simulink model "controlmodel"  (R2016a)
settings: Solver=ode45  StartTime=0.0  StopTime=12.0  RelTol=1e-3
values from neighbouring files (symbols this model uses):
  gainBFL = 1    [LoadModel_dampedTM.m]
  gainBFP = 1    [LoadModel_dampedTM.m]
  gainBFR = 1    [LoadModel_dampedTM.m]
  gainBFT = 1    [LoadModel_dampedTM.m]
  gainBFV = 1    [LoadModel_dampedTM.m]
  gainBFY = 1    [LoadModel_dampedTM.m]
  gainGASBF = 1    [LoadModel_dampedTM.m]
  gainGASF0 = 1    [LoadModel_dampedTM.m]
  gainGASF1 = 1    [LoadModel_dampedTM.m]
  gainGASF2 = 1    [LoadModel_dampedTM.m]
  gainGASF3 = 1    [LoadModel_dampedTM.m]
  gainIML = 1    [LoadModel_dampedTM.m]
  gainIMP = 1    [LoadModel_dampedTM.m]
  gainIMR = 1    [LoadModel_dampedTM.m]
  gainIMT = 1    [LoadModel_dampedTM.m]
  gainIMV = 1    [LoadModel_dampedTM.m]
  gainIMY = 1    [LoadModel_dampedTM.m]
  gainIPL = 1    [LoadModel_dampedTM.m]
  gainIPT = 1    [LoadModel_dampedTM.m]
  gainIPY = 1    [LoadModel_dampedTM.m]
  gainLOCK_IML = 1    [LoadModel_dampedTM.m]
  gainLOCK_IMP = 1    [LoadModel_dampedTM.m]
  gainLOCK_IMY = 1    [LoadModel_dampedTM.m]
  gainMNL = 1    [LoadModel_dampedTM.m]
  gainMNLOCK_L = 1    [LoadModel_dampedTM.m]
  gainMNLOCK_P = 1    [LoadModel_dampedTM.m]
  gainMNLOCK_Y = 1    [LoadModel_dampedTM.m]
  gainMNP = 1    [LoadModel_dampedTM.m]
  gainMNR = 1    [LoadModel_dampedTM.m]
  gainMNT = 1    [LoadModel_dampedTM.m]
  gainMNV = 1    [LoadModel_dampedTM.m]
  gainMNY = 1    [LoadModel_dampedTM.m]
  gainOL_MNP = 1    [LoadModel_dampedTM.m]
  gainOL_MNY = 1    [LoadModel_dampedTM.m]
  gainTML = 1    [LoadModel_dampedTM.m]
  gainTML_LOCK = 0    [LoadModel_dampedTM.m]
  gainTMOL_IML = 1    [LoadModel_dampedTM.m]
  gainTMOL_IMP = 1    [LoadModel_dampedTM.m]
  gainTMOL_IMY = 1    [LoadModel_dampedTM.m]
  gainTMOL_MNL = 1    [LoadModel_dampedTM.m]
  gainTMOL_MNP = 1    [LoadModel_dampedTM.m]
  gainTMOL_MNY = 1    [LoadModel_dampedTM.m]
  gainTMP = 1    [LoadModel_dampedTM.m]
  gainTMY = 1    [LoadModel_dampedTM.m]
  Kopt_angle = 0.1    [LoadModel_dampedTM.m]
  Kopt_len = 0.1    [LoadModel_dampedTM.m]
  optic = 'ETMX'    [LoadModel_dampedTM.m]
undefined symbols (not defined in the file or in its folder): cMat_BF, cMat_IM, cMat_MN, cMat_TM, Filt, gain_actBFGAS, gain_actBFL, gain_actBFP, gain_actBFR, gain_actBFT, gain_actBFV, gain_actBFY, gain_actF0GAS, gain_actF1GAS, gain_actF2GAS, gain_actF3GAS, gain_actIML, gain_actIMP, gain_actIMR, gain_actIMT, gain_actIMV, gain_actIMY, gain_actIPL, gain_actIPT, gain_actIPY, gain_actMNL, gain_actMNP, gain_actMNR, gain_actMNT, gain_actMNV, gain_actMNY, gain_actTML, gain_actTMP, gain_actTMY, SW, sys1
libraries: cstblocks x49, LiveParts x49
(part 2 of 3)

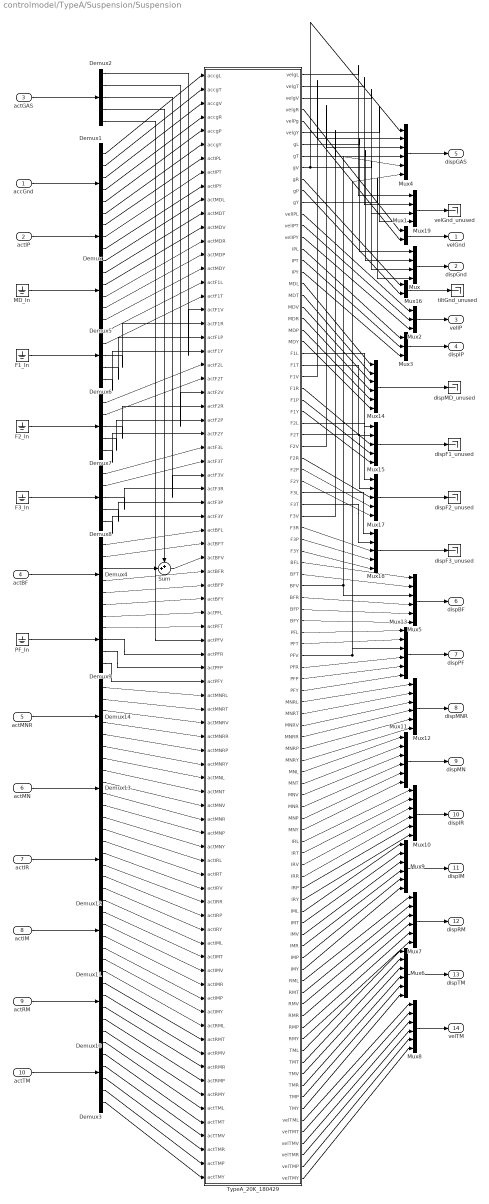
== system controlmodel/TypeA/Suspension/Suspension ==
  accGnd : Inport
  actIP : Inport  Port=2
  actGAS : Inport  Port=3
  actBF : Inport  Port=4
  actMNR : Inport  Port=5
  actMN : Inport  Port=6
  actIR : Inport  Port=7
  actIM : Inport  Port=8
  actRM : Inport  Port=9
  actTM : Inport  Port=10
  Demux : Demux  Outputs=3
  Demux{1,3..5,10..14} (9 alike) : Demux  Outputs=6
  Demux{2,6..9} (5 alike) : Demux  Outputs=5
  F1_In : Ground
  F2_In : Ground
  F3_In : Ground
  MD_In : Ground
  Mux : Mux
  Mux1 : Mux  Inputs=2
  Mux{4..14} (11 alike) : Mux  Inputs=6
  Mux15 : Mux  Inputs=5
  Mux16 : Mux  Inputs=2
  Mux17 : Mux  Inputs=5
  Mux18 : Mux  Inputs=5
  Mux19 : Mux
  Mux2 : Mux  Inputs=3
  Mux3 : Mux  Inputs=3
  PF_In : Ground
  Sum : Sum  Inputs=++|
  TypeA_20K_180429 : Subsystem
  dispF1_unused : Terminator
  dispF2_unused : Terminator
  dispF3_unused : Terminator
  dispMD_unused : Terminator
  tiltGnd_unused : Terminator
  velGnd_unused : Terminator
  velGnd : Outport
  dispGnd : Outport  Port=2
  velIP : Outport  Port=3
  dispIP : Outport  Port=4
  dispGAS : Outport  Port=5
  dispBF : Outport  Port=6
  dispPF : Outport  Port=7
  dispMNR : Outport  Port=8
  dispMN : Outport  Port=9
  dispIR : Outport  Port=10
  dispIM : Outport  Port=11
  dispRM : Outport  Port=12
  dispTM : Outport  Port=13
  velTM : Outport  Port=14
  wires:
  Mux/1 -> dispGnd/1
  Mux1/1 -> velGnd/1
  Mux2/1 -> velIP/1
  Mux3/1 -> dispIP/1
  Mux4/1 -> dispGAS/1
  Mux5/1 -> dispBF/1
  Mux6/1 -> dispTM/1
  actIP/1 -> Demux/1
  accGnd/1 -> Demux1/1
  actTM/1 -> Demux3/1
  Demux4/3 -> Sum/2
  Demux2/4 -> Sum/1
  Demux2/5 -> TypeA_20K_180429/42(actPFV)
  actBF/1 -> Demux4/1
  actGAS/1 -> Demux2/1
  Demux1/3 -> TypeA_20K_180429/3(accgV)
  Demux1/1 -> TypeA_20K_180429/1(accgL)
  Demux1/2 -> TypeA_20K_180429/2(accgT)
  Demux1/4 -> TypeA_20K_180429/4(accgR)
  Demux1/5 -> TypeA_20K_180429/5(accgP)
  Demux1/6 -> TypeA_20K_180429/6(accgY)
  Demux/1 -> TypeA_20K_180429/7(actIPL)
  Demux/2 -> TypeA_20K_180429/8(actIPT)
  Demux/3 -> TypeA_20K_180429/9(actIPY)
  MD_In/1 -> Demux5/1
  Demux5/1 -> TypeA_20K_180429/10(actMDL)
  Demux5/2 -> TypeA_20K_180429/11(actMDT)
  Demux5/3 -> TypeA_20K_180429/12(actMDV)
  Demux5/4 -> TypeA_20K_180429/13(actMDR)
  Demux5/5 -> TypeA_20K_180429/14(actMDP)
  Demux5/6 -> TypeA_20K_180429/15(actMDY)
  Demux2/1 -> TypeA_20K_180429/18(actF1V)
  Demux2/2 -> TypeA_20K_180429/24(actF2V)
  Demux2/3 -> TypeA_20K_180429/30(actF3V)
  Sum/1 -> TypeA_20K_180429/36(actBFV)
  F1_In/1 -> Demux6/1
  Demux6/2 -> TypeA_20K_180429/17(actF1T)
  Demux6/1 -> TypeA_20K_180429/16(actF1L)
  Demux6/5 -> TypeA_20K_180429/21(actF1Y)
  Demux6/3 -> TypeA_20K_180429/19(actF1R)
  Demux6/4 -> TypeA_20K_180429/20(actF1P)
  F2_In/1 -> Demux7/1
  Demux7/1 -> TypeA_20K_180429/22(actF2L)
  Demux7/2 -> TypeA_20K_180429/23(actF2T)
  Demux7/3 -> TypeA_20K_180429/25(actF2R)
  Demux7/4 -> TypeA_20K_180429/26(actF2P)
  Demux7/5 -> TypeA_20K_180429/27(actF2Y)
  F3_In/1 -> Demux8/1
  Demux8/2 -> TypeA_20K_180429/29(actF3T)
  Demux8/1 -> TypeA_20K_180429/28(actF3L)
  Demux8/5 -> TypeA_20K_180429/33(actF3Y)
  Demux8/4 -> TypeA_20K_180429/32(actF3P)
  Demux8/3 -> TypeA_20K_180429/31(actF3R)
  Demux4/1 -> TypeA_20K_180429/34(actBFL)
  Demux4/2 -> TypeA_20K_180429/35(actBFT)
  Demux4/4 -> TypeA_20K_180429/37(actBFR)
  Demux4/5 -> TypeA_20K_180429/38(actBFP)
  Demux4/6 -> TypeA_20K_180429/39(actBFY)
  PF_In/1 -> Demux9/1
  Demux9/1 -> TypeA_20K_180429/40(actPFL)
  Demux9/2 -> TypeA_20K_180429/41(actPFT)
  Demux9/4 -> TypeA_20K_180429/44(actPFP)
  Demux9/3 -> TypeA_20K_180429/43(actPFR)
  Demux9/5 -> TypeA_20K_180429/45(actPFY)
  actRM/1 -> Demux10/1
  actIM/1 -> Demux11/1
  actIR/1 -> Demux12/1
  actMN/1 -> Demux13/1
  actMNR/1 -> Demux14/1
  Demux14/4 -> TypeA_20K_180429/49(actMNRR)
  Demux14/5 -> TypeA_20K_180429/50(actMNRP)
  Demux14/6 -> TypeA_20K_180429/51(actMNRY)
  Demux14/1 -> TypeA_20K_180429/46(actMNRL)
  Demux14/2 -> TypeA_20K_180429/47(actMNRT)
  Demux14/3 -> TypeA_20K_180429/48(actMNRV)
  Demux13/2 -> TypeA_20K_180429/53(actMNT)
  Demux13/1 -> TypeA_20K_180429/52(actMNL)
  Demux13/3 -> TypeA_20K_180429/54(actMNV)
  Demux13/5 -> TypeA_20K_180429/56(actMNP)
  Demux13/4 -> TypeA_20K_180429/55(actMNR)
  Demux13/6 -> TypeA_20K_180429/57(actMNY)
  Demux12/6 -> TypeA_20K_180429/63(actIRY)
  Demux12/2 -> TypeA_20K_180429/59(actIRT)
  Demux12/5 -> TypeA_20K_180429/62(actIRP)
  Demux12/3 -> TypeA_20K_180429/60(actIRV)
  Demux12/4 -> TypeA_20K_180429/61(actIRR)
  Demux12/1 -> TypeA_20K_180429/58(actIRL)
  Demux11/2 -> TypeA_20K_180429/65(actIMT)
  Demux11/3 -> TypeA_20K_180429/66(actIMV)
  Demux11/5 -> TypeA_20K_180429/68(actIMP)
  Demux11/4 -> TypeA_20K_180429/67(actIMR)
  Demux11/1 -> TypeA_20K_180429/64(actIML)
  Demux11/6 -> TypeA_20K_180429/69(actIMY)
  Demux10/5 -> TypeA_20K_180429/74(actRMP)
  Demux10/6 -> TypeA_20K_180429/75(actRMY)
  Demux10/4 -> TypeA_20K_180429/73(actRMR)
  Demux10/3 -> TypeA_20K_180429/72(actRMV)
  Demux10/1 -> TypeA_20K_180429/70(actRML)
  Demux10/2 -> TypeA_20K_180429/71(actRMT)
  Demux3/3 -> TypeA_20K_180429/78(actTMV)
  Demux3/1 -> TypeA_20K_180429/76(actTML)
  Demux3/2 -> TypeA_20K_180429/77(actTMT)
  Demux3/4 -> TypeA_20K_180429/79(actTMR)
  Demux3/5 -> TypeA_20K_180429/80(actTMP)
  Demux3/6 -> TypeA_20K_180429/81(actTMY)
  Mux7/1 -> dispRM/1
  Mux8/1 -> velTM/1
  Mux9/1 -> dispIM/1
  Mux10/1 -> dispIR/1
  Mux11/1 -> dispMN/1
  Mux12/1 -> dispMNR/1
  Mux13/1 -> dispPF/1
  Mux14/1 -> dispMD_unused/1
  Mux15/1 -> dispF1_unused/1
  Mux16/1 -> tiltGnd_unused/1
  Mux17/1 -> dispF2_unused/1
  Mux18/1 -> dispF3_unused/1
  TypeA_20K_180429/4(velgR) -> Mux1/1
  TypeA_20K_180429/5(velPg) -> Mux1/2
  TypeA_20K_180429/8(gT) -> Mux/2
  TypeA_20K_180429/7(gL) -> Mux/1
  TypeA_20K_180429/9(gV) -> Mux/3, Mux4/1
  TypeA_20K_180429/11(gP) -> Mux16/2
  TypeA_20K_180429/10(gR) -> Mux16/1
  TypeA_20K_180429/12(gY) -> Mux/4
  TypeA_20K_180429/14(velIPT) -> Mux2/2
  TypeA_20K_180429/15(velIPY) -> Mux2/3
  TypeA_20K_180429/13(velIPL) -> Mux2/1
  TypeA_20K_180429/17(IPT) -> Mux3/2
  TypeA_20K_180429/16(IPL) -> Mux3/1
  TypeA_20K_180429/18(IPY) -> Mux3/3
  TypeA_20K_180429/19(MDL) -> Mux14/1
  TypeA_20K_180429/21(MDV) -> Mux14/3
  TypeA_20K_180429/20(MDT) -> Mux14/2
  TypeA_20K_180429/22(MDR) -> Mux14/4
  TypeA_20K_180429/23(MDP) -> Mux14/5
  TypeA_20K_180429/24(MDY) -> Mux14/6
  TypeA_20K_180429/27(F1V) -> Mux4/2
  TypeA_20K_180429/33(F2V) -> Mux4/3
  TypeA_20K_180429/39(F3V) -> Mux4/4
  TypeA_20K_180429/45(BFV) -> Mux4/5, Mux5/3
  TypeA_20K_180429/51(PFV) -> Mux4/6, Mux13/3
  TypeA_20K_180429/25(F1L) -> Mux15/1
  TypeA_20K_180429/26(F1T) -> Mux15/2
  TypeA_20K_180429/30(F1Y) -> Mux15/5
  TypeA_20K_180429/28(F1R) -> Mux15/3
  TypeA_20K_180429/29(F1P) -> Mux15/4
  TypeA_20K_180429/31(F2L) -> Mux17/1
  TypeA_20K_180429/32(F2T) -> Mux17/2
  TypeA_20K_180429/34(F2R) -> Mux17/3
  TypeA_20K_180429/36(F2Y) -> Mux17/5
  TypeA_20K_180429/35(F2P) -> Mux17/4
  TypeA_20K_180429/37(F3L) -> Mux18/1
  TypeA_20K_180429/38(F3T) -> Mux18/2
  TypeA_20K_180429/42(F3Y) -> Mux18/5
  TypeA_20K_180429/41(F3P) -> Mux18/4
  TypeA_20K_180429/40(F3R) -> Mux18/3
  TypeA_20K_180429/47(BFP) -> Mux5/5
  TypeA_20K_180429/48(BFY) -> Mux5/6
  TypeA_20K_180429/46(BFR) -> Mux5/4
  TypeA_20K_180429/44(BFT) -> Mux5/2
  TypeA_20K_180429/43(BFL) -> Mux5/1
  TypeA_20K_180429/54(PFY) -> Mux13/6
  TypeA_20K_180429/49(PFL) -> Mux13/1
  TypeA_20K_180429/50(PFT) -> Mux13/2
  TypeA_20K_180429/52(PFR) -> Mux13/4
  TypeA_20K_180429/53(PFP) -> Mux13/5
  TypeA_20K_180429/56(MNRT) -> Mux12/2
  TypeA_20K_180429/60(MNRY) -> Mux12/6
  TypeA_20K_180429/57(MNRV) -> Mux12/3
  TypeA_20K_180429/58(MNRR) -> Mux12/4
  TypeA_20K_180429/55(MNRL) -> Mux12/1
  TypeA_20K_180429/59(MNRP) -> Mux12/5
  TypeA_20K_180429/64(MNR) -> Mux11/4
  TypeA_20K_180429/61(MNL) -> Mux11/1
  TypeA_20K_180429/63(MNV) -> Mux11/3
  TypeA_20K_180429/62(MNT) -> Mux11/2
  TypeA_20K_180429/66(MNY) -> Mux11/6
  TypeA_20K_180429/65(MNP) -> Mux11/5
  TypeA_20K_180429/71(IRP) -> Mux10/5
  TypeA_20K_180429/69(IRV) -> Mux10/3
  TypeA_20K_180429/72(IRY) -> Mux10/6
  TypeA_20K_180429/70(IRR) -> Mux10/4
  TypeA_20K_180429/68(IRT) -> Mux10/2
  TypeA_20K_180429/67(IRL) -> Mux10/1
  TypeA_20K_180429/73(IML) -> Mux9/1
  TypeA_20K_180429/75(IMV) -> Mux9/3
  TypeA_20K_180429/74(IMT) -> Mux9/2
  TypeA_20K_180429/76(IMR) -> Mux9/4
  TypeA_20K_180429/77(IMP) -> Mux9/5
  TypeA_20K_180429/78(IMY) -> Mux9/6
  TypeA_20K_180429/83(RMP) -> Mux7/5
  TypeA_20K_180429/84(RMY) -> Mux7/6
  TypeA_20K_180429/79(RML) -> Mux7/1
  TypeA_20K_180429/81(RMV) -> Mux7/3
  TypeA_20K_180429/80(RMT) -> Mux7/2
  TypeA_20K_180429/82(RMR) -> Mux7/4
  TypeA_20K_180429/85(TML) -> Mux6/1
  TypeA_20K_180429/86(TMT) -> Mux6/2
  TypeA_20K_180429/88(TMR) -> Mux6/4
  TypeA_20K_180429/87(TMV) -> Mux6/3
  TypeA_20K_180429/89(TMP) -> Mux6/5
  TypeA_20K_180429/90(TMY) -> Mux6/6
  TypeA_20K_180429/93(velTMV) -> Mux8/3
  TypeA_20K_180429/94(velTMR) -> Mux8/4
  TypeA_20K_180429/96(velTMY) -> Mux8/6
  TypeA_20K_180429/91(velTML) -> Mux8/1
  TypeA_20K_180429/95(velTMP) -> Mux8/5
  TypeA_20K_180429/92(velTMT) -> Mux8/2
  Mux19/1 -> velGnd_unused/1
  TypeA_20K_180429/1(velgL) -> Mux19/1
  TypeA_20K_180429/2(velgT) -> Mux19/2
  TypeA_20K_180429/3(velgV) -> Mux19/3
  TypeA_20K_180429/6(velgY) -> Mux19/4

== system controlmodel/TypeA/Suspension/aMatrix_BF ==
  aMat_in : Inport
  cMat_BF : Constant  Value=cMat_BF  VectorParams1D=off
  coupling_BF : Product  Multiplication=Matrix(*)
  actBF : Outport
  wires:
  coupling_BF/1 -> actBF/1
  aMat_in/1 -> coupling_BF/2
  cMat_BF/1 -> coupling_BF/1

== system controlmodel/TypeA/Suspension/aMatrix_GAS ==
  aMat_in : Inport
  Add{1..4} (4 alike) : Sum  Inputs=+-
  Demux4 : Demux  Outputs=5
  Mux3 : Mux  Inputs=5
  actGAS : Outport
  wires:
  aMat_in/1 -> Demux4/1
  Mux3/1 -> actGAS/1
  Add1/1 -> Mux3/1
  Add2/1 -> Mux3/2
  Demux4/3 -> Add3/1, Add2/2
  Demux4/2 -> Add1/2, Add2/1
  Demux4/1 -> Add1/1
  Demux4/5 -> Mux3/5, Add4/2
  Add4/1 -> Mux3/4
  Add3/1 -> Mux3/3
  Demux4/4 -> Add3/2, Add4/1

== system controlmodel/TypeA/Suspension/aMatrix_IM ==
  aMat_in : Inport
  Gain : Gain  Gain=-1
  cMat_IM : Constant  Value=cMat_IM  VectorParams1D=off
  coupling_IM : Product  Multiplication=Matrix(*)
  actIR : Outport
  actIM : Outport  Port=2
  wires:
  coupling_IM/1 -> actIM/1, Gain/1
  aMat_in/1 -> coupling_IM/2
  cMat_IM/1 -> coupling_IM/1
  Gain/1 -> actIR/1

== system controlmodel/TypeA/Suspension/aMatrix_MN ==
  aMat_in : Inport
  Gain : Gain  Gain=-1
  cMat_MN : Constant  Value=cMat_MN  VectorParams1D=off
  coupling_MN : Product  Multiplication=Matrix(*)
  actMNR : Outport
  actMN : Outport  Port=2
  wires:
  coupling_MN/1 -> actMN/1, Gain/1
  aMat_in/1 -> coupling_MN/2
  cMat_MN/1 -> coupling_MN/1
  Gain/1 -> actMNR/1

== system controlmodel/TypeA/Suspension/aMatrix_TM ==
  aMat_in : Inport
  Demux : Demux  Outputs=3
  Demux1 : Demux  Outputs=3
  Gain : Gain  Gain=-1
  Ground{,1..5} (6 alike) : Ground
  Mux : Mux  Inputs=6
  Mux1 : Mux  Inputs=6
  cMat_TM : Constant  Value=cMat_TM  VectorParams1D=off
  coupling_TM : Product  Multiplication=Matrix(*)
  actRM : Outport
  actTM : Outport  Port=2
  wires:
  coupling_TM/1 -> Demux1/1, Gain/1
  aMat_in/1 -> coupling_TM/2  "3DoF"
  cMat_TM/1 -> coupling_TM/1
  Gain/1 -> Demux/1
  Demux/1 -> Mux/1
  Demux/2 -> Mux/5
  Demux/3 -> Mux/6
  Demux1/1 -> Mux1/1
  Demux1/3 -> Mux1/6
  Demux1/2 -> Mux1/5
  Ground/1 -> Mux/2
  Ground1/1 -> Mux/3
  Ground2/1 -> Mux/4
  Ground4/1 -> Mux1/3
  Ground3/1 -> Mux1/2
  Ground5/1 -> Mux1/4
  Mux/1 -> actRM/1  "6DoF"
  Mux1/1 -> actTM/1  "6DoF"

== system controlmodel/TypeA/Suspension/sMatrix_BF_LVDT ==
  dispGnd : Inport
  dispBF : Inport  Port=2
  Add2 : Sum  Inputs=-+
  Demux : Demux
  Ground : Ground
  Ground1 : Ground
  Mux : Mux  Inputs=6
  BF_LVDT : Outport
  wires:
  Add2/1 -> BF_LVDT/1  "6DoF"
  dispBF/1 -> Add2/2  "6DoF"
  dispGnd/1 -> Demux/1  "4DoF"
  Demux/1 -> Mux/1  "L"
  Demux/2 -> Mux/2  "T"
  Demux/3 -> Mux/3  "V"
  Demux/4 -> Mux/6  "Y"
  Ground/1 -> Mux/4  "R"
  Ground1/1 -> Mux/5  "P"
  Mux/1 -> Add2/1

== system controlmodel/TypeA/Suspension/sMatrix_GAS_LVDT ==
  dispGAS : Inport
  Add{1..5} (5 alike) : Sum  Inputs=-+
  Demux4 : Demux  Outputs=6
  Mux3 : Mux  Inputs=5
  GAS_LVDT : Outport
  wires:
  dispGAS/1 -> Demux4/1
  Demux4/1 -> Add2/1  "VGnd = IPV"
  Demux4/2 -> Add1/1, Add2/2  "VF1"
  Demux4/3 -> Add1/2, Add3/1  "VF2"
  Demux4/4 -> Add4/1, Add3/2  "VF3"
  Add2/1 -> Mux3/1  "GASF0"
  Add1/1 -> Mux3/2  "GASF1"
  Add3/1 -> Mux3/3  "GASF2"
  Mux3/1 -> GAS_LVDT/1
  Demux4/5 -> Add5/1, Add4/2  "VBF"
  Demux4/6 -> Add5/2  "VPF"
  Add4/1 -> Mux3/4  "GASF3"
  Add5/1 -> Mux3/5  "GASBF"

== system controlmodel/TypeA/Suspension/sMatrix_IM_PS ==
  dispIR : Inport
  dispIM : Inport  Port=2
  Add2 : Sum  Inputs=-+
  IM_PS : Outport
  wires:
  Add2/1 -> IM_PS/1
  dispIM/1 -> Add2/2
  dispIR/1 -> Add2/1

== system controlmodel/TypeA/Suspension/sMatrix_IP_LVDT ==
  dispGnd : Inport
  dispIP : Inport  Port=2
  Add2 : Sum  Inputs=-+
  Demux : Demux
  Mux : Mux  Inputs=3
  Terminator : Terminator
  IP_LVDT : Outport
  wires:
  Add2/1 -> IP_LVDT/1
  dispIP/1 -> Add2/2
  dispGnd/1 -> Demux/1
  Demux/1 -> Mux/1  "L"
  Demux/2 -> Mux/2  "T"
  Demux/4 -> Mux/3  "Y"
  Demux/3 -> Terminator/1  "V"
  Mux/1 -> Add2/1

== system controlmodel/TypeA/Suspension/sMatrix_MN_OpLev ==
  dispMN : Inport
  Demux4 : Demux  Outputs=6
  Mux3 : Mux  Inputs=3
  dispMNL : Terminator
  dispMNT : Terminator
  dispMNV : Terminator
  MN_OpLev : Outport
  wires:
  dispMN/1 -> Demux4/1
  Mux3/1 -> MN_OpLev/1
  Demux4/1 -> dispMNL/1
  Demux4/2 -> dispMNT/1
  Demux4/3 -> dispMNV/1
  Demux4/4 -> Mux3/1
  Demux4/5 -> Mux3/2
  Demux4/6 -> Mux3/3

== system controlmodel/TypeA/Suspension/sMatrix_MN_PS ==
  dispMNR : Inport
  dispMN : Inport  Port=2
  Add2 : Sum  Inputs=-+
  MN_PS : Outport
  wires:
  Add2/1 -> MN_PS/1
  dispMN/1 -> Add2/2
  dispMNR/1 -> Add2/1

== system controlmodel/TypeA/Suspension/sMatrix_PF_OpLev ==
  dispPF : Inport
  Demux4 : Demux  Outputs=6
  Mux3 : Mux  Inputs=3
  dispLPF : Terminator
  dispTPF : Terminator
  dispVPF : Terminator
  OpLev_PF : Outport
  wires:
  dispPF/1 -> Demux4/1
  Mux3/1 -> OpLev_PF/1
  Demux4/1 -> dispLPF/1
  Demux4/2 -> dispTPF/1
  Demux4/3 -> dispVPF/1
  Demux4/4 -> Mux3/1
  Demux4/5 -> Mux3/2
  Demux4/6 -> Mux3/3

== system controlmodel/TypeA/Suspension/sMatrix_TM_OpLev ==
  dispTM : Inport
  dispGND : Inport  Port=2
  Add : Sum  Inputs=-+
  Demux : Demux
  Demux4 : Demux  Outputs=6
  Mux3 : Mux  Inputs=3
  dispTMR : Terminator
  dispTMT{,1..3} (4 alike) : Terminator
  dispTMV : Terminator
  TM_OpLev : Outport
  wires:
  dispTM/1 -> Demux4/1
  Mux3/1 -> TM_OpLev/1
  Demux4/2 -> dispTMT/1
  Demux4/3 -> dispTMV/1
  Demux4/4 -> dispTMR/1
  Demux4/5 -> Mux3/2
  Demux4/6 -> Mux3/3
  Demux/1 -> Add/1
  dispGND/1 -> Demux/1
  Demux/2 -> dispTMT1/1
  Demux/3 -> dispTMT2/1
  Demux/4 -> dispTMT3/1
  Demux4/1 -> Add/2
  Add/1 -> Mux3/1

== system controlmodel/TypeA/Suspension/sMatrix_TM_PS ==
  dispRM : Inport
  dispTM : Inport  Port=2
  Add2 : Sum  Inputs=-+
  Demux : Demux  Outputs=6
  Demux1 : Demux  Outputs=6
  Mux : Mux  Inputs=3
  Mux1 : Mux  Inputs=3
  Terminator{,1..5} (6 alike) : Terminator
  TM_PS : Outport
  wires:
  Add2/1 -> TM_PS/1  "(L, P, Y)"
  dispRM/1 -> Demux/1
  dispTM/1 -> Demux1/1
  Demux/1 -> Mux/1  "L"
  Demux/5 -> Mux/2  "P"
  Demux/6 -> Mux/3  "Y"
  Demux1/1 -> Mux1/1  "L"
  Demux1/5 -> Mux1/2  "P"
  Demux1/6 -> Mux1/3  "Y"
  Mux/1 -> Add2/1
  Mux1/1 -> Add2/2
  Demux/2 -> Terminator/1  "T"
  Demux/4 -> Terminator2/1  "R"
  Demux/3 -> Terminator1/1  "V"
  Demux1/4 -> Terminator5/1  "R"
  Demux1/2 -> Terminator3/1  "T"
  Demux1/3 -> Terminator4/1  "V"

== system controlmodel/TypeA/Controller/BFservo/Servo_LBF ==
  In : Inport
  BF_DAMP_L : cstblocks/LTI System  sys=Filt('BF_DAMP_L')  IC=[]
  K1:VIS-OPTIC_BF_DAMP_L : LiveParts/LiveFilter  Tag=LiveFilter  par=Filt_BF_DAMP_L  prefix=['K1:VIS-',optic,'_BF_DAMP_L']  site='kamioka'  feModel=['K1VIS',optic,'T']  fmName=[optic,'_BF_DAMP_L']  flexTf=on  viewGui=off
      settings: AttributesFormatString=%<Tag>
  Out : Outport
  wires:
  In/1 -> BF_DAMP_L/1
  BF_DAMP_L/1 -> Out/1

== system controlmodel/TypeA/Controller/BFservo/Servo_PBF ==
  In : Inport
  BF_DAMP_P : cstblocks/LTI System  sys=Filt('BF_DAMP_P')  IC=[]
  K1:VIS-OPTIC_BF_DAMP_P : LiveParts/LiveFilter  Tag=LiveFilter  par=Filt_BF_DAMP_P  prefix=['K1:VIS-',optic,'_BF_DAMP_P']  site='kamioka'  feModel=['K1VIS',optic,'T']  fmName=[optic,'_BF_DAMP_P']  flexTf=on  viewGui=off
      settings: AttributesFormatString=%<Tag>
  Out : Outport
  wires:
  In/1 -> BF_DAMP_P/1
  BF_DAMP_P/1 -> Out/1

== system controlmodel/TypeA/Controller/BFservo/Servo_RBF ==
  In : Inport
  BF_DAMP_R : cstblocks/LTI System  sys=Filt('BF_DAMP_R')  IC=[]
  K1:VIS-OPTIC_BF_DAMP_R : LiveParts/LiveFilter  Tag=LiveFilter  par=Filt_BF_DAMP_R  prefix=['K1:VIS-',optic,'_BF_DAMP_R']  site='kamioka'  feModel=['K1VIS',optic,'T']  fmName=[optic,'_BF_DAMP_R']  flexTf=on  viewGui=off
      settings: AttributesFormatString=%<Tag>
  Out : Outport
  wires:
  In/1 -> BF_DAMP_R/1
  BF_DAMP_R/1 -> Out/1

== system controlmodel/TypeA/Controller/BFservo/Servo_TBF ==
  In : Inport
  BF_DAMP_T : cstblocks/LTI System  sys=Filt('BF_DAMP_T')  IC=[]
  K1:VIS-OPTIC_BF_DAMP_T : LiveParts/LiveFilter  Tag=LiveFilter  par=Filt_BF_DAMP_T  prefix=['K1:VIS-',optic,'_BF_DAMP_T']  site='kamioka'  feModel=['K1VIS',optic,'T']  fmName=[optic,'_BF_DAMP_T']  flexTf=on  viewGui=off
      settings: AttributesFormatString=%<Tag>
  Out : Outport
  wires:
  In/1 -> BF_DAMP_T/1
  BF_DAMP_T/1 -> Out/1

== system controlmodel/TypeA/Controller/BFservo/Servo_VBF ==
  In : Inport
  BF_DAMP_V : cstblocks/LTI System  sys=Filt('BF_DAMP_V')  IC=[]
  K1:VIS-OPTIC_BF_DAMP_V : LiveParts/LiveFilter  Tag=LiveFilter  par=Filt_BF_DAMP_V  prefix=['K1:VIS-',optic,'_BF_DAMP_V']  site='kamioka'  feModel=['K1VIS',optic,'T']  fmName=[optic,'_BF_DAMP_V']  flexTf=on  viewGui=off
      settings: AttributesFormatString=%<Tag>
  Out : Outport
  wires:
  In/1 -> BF_DAMP_V/1
  BF_DAMP_V/1 -> Out/1

== system controlmodel/TypeA/Controller/BFservo/Servo_YBF ==
  In : Inport
  BF_DAMP_Y : cstblocks/LTI System  sys=Filt('BF_DAMP_Y')  IC=[]
  K1:VIS-OPTIC_BF_DAMP_Y : LiveParts/LiveFilter  Tag=LiveFilter  par=Filt_BF_DAMP_Y  prefix=['K1:VIS-',optic,'_BF_DAMP_Y']  site='kamioka'  feModel=['K1VIS',optic,'T']  fmName=[optic,'_BF_DAMP_Y']  flexTf=on  viewGui=off
      settings: AttributesFormatString=%<Tag>
  Out : Outport
  wires:
  In/1 -> BF_DAMP_Y/1
  BF_DAMP_Y/1 -> Out/1

== system controlmodel/TypeA/Controller/GASservo/Servo_GASBF ==
  In : Inport
  BF_DAMP_GAS : cstblocks/LTI System  sys=Filt('BF_DAMP_GAS')  IC=[]
  K1:VIS-OPTIC_BF_DAMP_GAS : LiveParts/LiveFilter  Tag=LiveFilter  par=Filt_BF_DAMP_GAS  prefix=['K1:VIS-',optic,'_BF_DAMP_GAS']  site='kamioka'  feModel=['K1VIS',optic,'T']  fmName=[optic,'_BF_DAMP_GAS']  flexTf=on  viewGui=off
      settings: AttributesFormatString=%<Tag>
  Out : Outport
  wires:
  In/1 -> BF_DAMP_GAS/1
  BF_DAMP_GAS/1 -> Out/1

== system controlmodel/TypeA/Controller/GASservo/Servo_GASF0 ==
  In : Inport
  F0_DAMP_GAS : cstblocks/LTI System  sys=Filt('F0_DAMP_GAS')  IC=[]
  K1:VIS-OPTIC_F0_DAMP_GAS : LiveParts/LiveFilter  Tag=LiveFilter  par=Filt_F0_DAMP_GAS  prefix=['K1:VIS-',optic,'_F0_DAMP_GAS']  site='kamioka'  feModel=['K1VIS',optic,'T']  fmName=[optic,'_F0_DAMP_GAS']  flexTf=on  viewGui=off
      settings: AttributesFormatString=%<Tag>
  Out : Outport
  wires:
  In/1 -> F0_DAMP_GAS/1
  F0_DAMP_GAS/1 -> Out/1

== system controlmodel/TypeA/Controller/GASservo/Servo_GASF1 ==
  In : Inport
  F1_DAMP_GAS : cstblocks/LTI System  sys=Filt('F1_DAMP_GAS')  IC=[]
  K1:VIS-OPTIC_F1_DAMP_GAS : LiveParts/LiveFilter  Tag=LiveFilter  par=Filt_F1_DAMP_GAS  prefix=['K1:VIS-',optic,'_F1_DAMP_GAS']  site='kamioka'  feModel=['K1VIS',optic,'T']  fmName=[optic,'_F1_DAMP_GAS']  flexTf=on  viewGui=off
      settings: AttributesFormatString=%<Tag>
  Out : Outport
  wires:
  In/1 -> F1_DAMP_GAS/1
  F1_DAMP_GAS/1 -> Out/1

== system controlmodel/TypeA/Controller/GASservo/Servo_GASF2 ==
  In : Inport
  F2_DAMP_GAS : cstblocks/LTI System  sys=Filt('F2_DAMP_GAS')  IC=[]
  K1:VIS-OPTIC_F2_DAMP_GAS : LiveParts/LiveFilter  Tag=LiveFilter  par=Filt_F2_DAMP_GAS  prefix=['K1:VIS-',optic,'_F2_DAMP_GAS']  site='kamioka'  feModel=['K1VIS',optic,'T']  fmName=[optic,'_F2_DAMP_GAS']  flexTf=on  viewGui=off
      settings: AttributesFormatString=%<Tag>
  Out : Outport
  wires:
  In/1 -> F2_DAMP_GAS/1
  F2_DAMP_GAS/1 -> Out/1

== system controlmodel/TypeA/Controller/GASservo/Servo_GASF3 ==
  In : Inport
  F3_DAMP_GAS : cstblocks/LTI System  sys=Filt('F3_DAMP_GAS')  IC=[]
  K1:VIS-OPTIC_F3_DAMP_GAS : LiveParts/LiveFilter  Tag=LiveFilter  par=Filt_F3_DAMP_GAS  prefix=['K1:VIS-',optic,'_F3_DAMP_GAS']  site='kamioka'  feModel=['K1VIS',optic,'T']  fmName=[optic,'_F3_DAMP_GAS']  flexTf=on  viewGui=off
      settings: AttributesFormatString=%<Tag>
  Out : Outport
  wires:
  In/1 -> F3_DAMP_GAS/1
  F3_DAMP_GAS/1 -> Out/1

== system controlmodel/TypeA/Controller/IMservo/Damp_LIM ==
  In : Inport
  IM_PSDAMP_L : cstblocks/LTI System  sys=Filt('IM_PSDAMP_L')  IC=[]
  K1:VIS-OPTIC_IM_PSDAMP_L : LiveParts/LiveFilter  Tag=LiveFilter  par=Filt_IM_PSDAMP_L  prefix=['K1:VIS-',optic,'_IM_PSDAMP_L']  site='kamioka'  feModel=['K1VIS',optic,'P']  fmName=[optic,'_IM_PSDAMP_L']  flexTf=on  viewGui=off
      settings: AttributesFormatString=%<Tag>
  Out : Outport
  wires:
  In/1 -> IM_PSDAMP_L/1
  IM_PSDAMP_L/1 -> Out/1

== system controlmodel/TypeA/Controller/IMservo/Damp_PIM ==
  In : Inport
  IM_PSDAMP_P : cstblocks/LTI System  sys=Filt('IM_PSDAMP_P')  IC=[]
  K1:VIS-OPTIC_IM_PSDAMP_P : LiveParts/LiveFilter  Tag=LiveFilter  par=Filt_IM_PSDAMP_P  prefix=['K1:VIS-',optic,'_IM_PSDAMP_P']  site='kamioka'  feModel=['K1VIS',optic,'P']  fmName=[optic,'_IM_PSDAMP_P']  flexTf=on  viewGui=off
      settings: AttributesFormatString=%<Tag>
  Out : Outport
  wires:
  In/1 -> IM_PSDAMP_P/1
  IM_PSDAMP_P/1 -> Out/1

== system controlmodel/TypeA/Controller/IMservo/Damp_RIM ==
  In : Inport
  IM_PSDAMP_R : cstblocks/LTI System  sys=Filt('IM_PSDAMP_R')  IC=[]
  K1:VIS-OPTIC_IM_PSDAMP_R : LiveParts/LiveFilter  Tag=LiveFilter  par=Filt_IM_PSDAMP_R  prefix=['K1:VIS-',optic,'_IM_PSDAMP_R']  site='kamioka'  feModel=['K1VIS',optic,'P']  fmName=[optic,'_IM_PSDAMP_R']  flexTf=on  viewGui=off
      settings: AttributesFormatString=%<Tag>
  Out : Outport
  wires:
  In/1 -> IM_PSDAMP_R/1
  IM_PSDAMP_R/1 -> Out/1

== system controlmodel/TypeA/Controller/IMservo/Damp_TIM ==
  In : Inport
  IM_PSDAMP_T : cstblocks/LTI System  sys=Filt('IM_PSDAMP_T')  IC=[]
  K1:VIS-OPTIC_IM_PSDAMP_T : LiveParts/LiveFilter  Tag=LiveFilter  par=Filt_IM_PSDAMP_T  prefix=['K1:VIS-',optic,'_IM_PSDAMP_T']  site='kamioka'  feModel=['K1VIS',optic,'P']  fmName=[optic,'_IM_PSDAMP_T']  flexTf=on  viewGui=off
      settings: AttributesFormatString=%<Tag>
  Out : Outport
  wires:
  In/1 -> IM_PSDAMP_T/1
  IM_PSDAMP_T/1 -> Out/1

== system controlmodel/TypeA/Controller/IMservo/Damp_VIM ==
  In : Inport
  IM_PSDAMP_V : cstblocks/LTI System  sys=Filt('IM_PSDAMP_V')  IC=[]
  K1:VIS-OPTIC_IM_PSDAMP_V : LiveParts/LiveFilter  Tag=LiveFilter  par=Filt_IM_PSDAMP_V  prefix=['K1:VIS-',optic,'_IM_PSDAMP_V']  site='kamioka'  feModel=['K1VIS',optic,'P']  fmName=[optic,'_IM_PSDAMP_V']  flexTf=on  viewGui=off
      settings: AttributesFormatString=%<Tag>
  Out : Outport
  wires:
  In/1 -> IM_PSDAMP_V/1
  IM_PSDAMP_V/1 -> Out/1

== system controlmodel/TypeA/Controller/IMservo/Damp_YIM ==
  In : Inport
  IM_PSDAMP_Y : cstblocks/LTI System  sys=Filt('IM_PSDAMP_Y')  IC=[]
  K1:VIS-OPTIC_IM_PSDAMP_Y : LiveParts/LiveFilter  Tag=LiveFilter  par=Filt_IM_PSDAMP_Y  prefix=['K1:VIS-',optic,'_IM_PSDAMP_Y']  site='kamioka'  feModel=['K1VIS',optic,'P']  fmName=[optic,'_IM_PSDAMP_Y']  flexTf=on  viewGui=off
      settings: AttributesFormatString=%<Tag>
  Out : Outport
  wires:
  In/1 -> IM_PSDAMP_Y/1
  IM_PSDAMP_Y/1 -> Out/1

== system controlmodel/TypeA/Controller/IMservo/IMLOCK_L ==
  In : Inport
  IM_LOCK_L : cstblocks/LTI System  sys=Filt('IM_LOCK_L')  IC=[]
  K1:VIS-OPTIC_IM_LOCK_L : LiveParts/LiveFilter  Tag=LiveFilter  par=Filt_IM_LOCK_L  prefix=['K1:VIS-',optic,'_IM_LOCK_L']  site='kamioka'  feModel=['K1VIS',optic,'P']  fmName=[optic,'_IM_LOCK_L']  flexTf=on  viewGui=off
      settings: AttributesFormatString=%<Tag>
  Out : Outport
  wires:
  In/1 -> IM_LOCK_L/1
  IM_LOCK_L/1 -> Out/1

== system controlmodel/TypeA/Controller/IMservo/IMLOCK_P ==
  In : Inport
  IM_LOCK_P : cstblocks/LTI System  sys=Filt('IM_LOCK_P')  IC=[]
  K1:VIS-OPTIC_IM_LOCK_P : LiveParts/LiveFilter  Tag=LiveFilter  par=Filt_IM_LOCK_P  prefix=['K1:VIS-',optic,'_IM_LOCK_P']  site='kamioka'  feModel=['K1VIS',optic,'P']  fmName=[optic,'_IM_LOCK_P']  flexTf=on  viewGui=off
      settings: AttributesFormatString=%<Tag>
  Out : Outport
  wires:
  In/1 -> IM_LOCK_P/1
  IM_LOCK_P/1 -> Out/1

== system controlmodel/TypeA/Controller/IMservo/IMLOCK_Y ==
  In : Inport
  IM_LOCK_Y : cstblocks/LTI System  sys=Filt('IM_LOCK_Y')  IC=[]
  K1:VIS-OPTIC_IM_LOCK_Y : LiveParts/LiveFilter  Tag=LiveFilter  par=Filt_IM_LOCK_Y  prefix=['K1:VIS-',optic,'_IM_LOCK_Y']  site='kamioka'  feModel=['K1VIS',optic,'P']  fmName=[optic,'_IM_LOCK_Y']  flexTf=on  viewGui=off
      settings: AttributesFormatString=%<Tag>
  Out : Outport
  wires:
  In/1 -> IM_LOCK_Y/1
  IM_LOCK_Y/1 -> Out/1

== system controlmodel/TypeA/Controller/IMservo/TMOLDamp_LIM ==
  In : Inport
  IM_TMOLDAMP_L : cstblocks/LTI System  sys=Filt('IM_TMOLDAMP_L')  IC=[]
  K1:VIS-OPTIC_IM_TMOLDAMP_L : LiveParts/LiveFilter  Tag=LiveFilter  par=Filt_IM_TMOLDAMP_L  prefix=['K1:VIS-',optic,'_IM_TMOLDAMP_L']  site='kamioka'  feModel=['K1VIS',optic,'P']  fmName=[optic,'_IM_TMOLDAMP_L']  flexTf=on  viewGui=off
      settings: AttributesFormatString=%<Tag>
  Out : Outport
  wires:
  In/1 -> IM_TMOLDAMP_L/1
  IM_TMOLDAMP_L/1 -> Out/1

== system controlmodel/TypeA/Controller/IMservo/TMOLDamp_PIM ==
  In : Inport
  IM_TMOLDAMP_P : cstblocks/LTI System  sys=Filt('IM_TMOLDAMP_P')  IC=[]
  K1:VIS-OPTIC_IM_TMOLDAMP_P : LiveParts/LiveFilter  Tag=LiveFilter  par=Filt_IM_TMOLDAMP_P  prefix=['K1:VIS-',optic,'_IM_TMOLDAMP_P']  site='kamioka'  feModel=['K1VIS',optic,'P']  fmName=[optic,'_IM_TMOLDAMP_P']  flexTf=on  viewGui=off
      settings: AttributesFormatString=%<Tag>
  Out : Outport
  wires:
  In/1 -> IM_TMOLDAMP_P/1
  IM_TMOLDAMP_P/1 -> Out/1

== system controlmodel/TypeA/Controller/IMservo/TMOLDamp_YIM ==
  In : Inport
  IM_TMOLDAMP_Y : cstblocks/LTI System  sys=Filt('IM_TMOLDAMP_Y')  IC=[]
  K1:VIS-OPTIC_IM_TMOLDAMP_Y : LiveParts/LiveFilter  Tag=LiveFilter  par=Filt_IM_TMOLDAMP_Y  prefix=['K1:VIS-',optic,'_IM_TMOLDAMP_Y']  site='kamioka'  feModel=['K1VIS',optic,'P']  fmName=[optic,'_IM_TMOLDAMP_Y']  flexTf=on  viewGui=off
      settings: AttributesFormatString=%<Tag>
  Out : Outport
  wires:
  In/1 -> IM_TMOLDAMP_Y/1
  IM_TMOLDAMP_Y/1 -> Out/1

== system controlmodel/TypeA/Controller/IPservo/Servo_LIP ==
  In : Inport
  IP_DAMP_L : cstblocks/LTI System  sys=Filt('IP_DAMP_L')  IC=[]
  K1:VIS-OPTIC_IP_DAMP_L : LiveParts/LiveFilter  Tag=LiveFilter  par=Filt_IP_DAMP_L  prefix=['K1:VIS-',optic,'_IP_DAMP_L']  site='kamioka'  feModel=['K1VIS',optic,'T']  fmName=[optic,'_IP_DAMP_L']  flexTf=on  viewGui=off
      settings: AttributesFormatString=%<Tag>
  Out : Outport
  wires:
  In/1 -> IP_DAMP_L/1
  IP_DAMP_L/1 -> Out/1

== system controlmodel/TypeA/Controller/IPservo/Servo_TIP ==
  In : Inport
  IP_DAMP_T : cstblocks/LTI System  sys=Filt('IP_DAMP_T')  IC=[]
  K1:VIS-OPTIC_IP_DAMP_T : LiveParts/LiveFilter  Tag=LiveFilter  par=Filt_IP_DAMP_T  prefix=['K1:VIS-',optic,'_IP_DAMP_T']  site='kamioka'  feModel=['K1VIS',optic,'T']  fmName=[optic,'_IP_DAMP_T']  flexTf=on  viewGui=off
      settings: AttributesFormatString=%<Tag>
  Out : Outport
  wires:
  In/1 -> IP_DAMP_T/1
  IP_DAMP_T/1 -> Out/1

== system controlmodel/TypeA/Controller/IPservo/Servo_YIP ==
  In : Inport
  IP_DAMP_Y : cstblocks/LTI System  sys=Filt('IP_DAMP_Y')  IC=[]
  K1:VIS-OPTIC_IP_DAMP_Y : LiveParts/LiveFilter  Tag=LiveFilter  par=Filt_IP_DAMP_Y  prefix=['K1:VIS-',optic,'_IP_DAMP_Y']  site='kamioka'  feModel=['K1VIS',optic,'T']  fmName=[optic,'_IP_DAMP_Y']  flexTf=on  viewGui=off
      settings: AttributesFormatString=%<Tag>
  Out : Outport
  wires:
  In/1 -> IP_DAMP_Y/1
  IP_DAMP_Y/1 -> Out/1

== system controlmodel/TypeA/Controller/MNservo/Damp_LMN ==
  In : Inport
  K1:VIS-OPTIC_MN_PSDAMP_L : LiveParts/LiveFilter  Tag=LiveFilter  par=Filt_MN_PSDAMP_L  prefix=['K1:VIS-',optic,'_MN_PSDAMP_L']  site='kamioka'  feModel=['K1VIS',optic,'P']  fmName=[optic,'_MN_PSDAMP_L']  flexTf=on  viewGui=off
      settings: AttributesFormatString=%<Tag>
  MN_PSDAMP_L : cstblocks/LTI System  sys=Filt('MN_PSDAMP_L')  IC=[]
  Out : Outport
  wires:
  In/1 -> MN_PSDAMP_L/1
  MN_PSDAMP_L/1 -> Out/1

== system controlmodel/TypeA/Controller/MNservo/Damp_PMN ==
  In : Inport
  K1:VIS-OPTIC_MN_PSDAMP_P : LiveParts/LiveFilter  Tag=LiveFilter  par=Filt_MN_PSDAMP_P  prefix=['K1:VIS-',optic,'_MN_PSDAMP_P']  site='kamioka'  feModel=['K1VIS',optic,'P']  fmName=[optic,'_MN_PSDAMP_P']  flexTf=on  viewGui=off
      settings: AttributesFormatString=%<Tag>
  MN_PSDAMP_P : cstblocks/LTI System  sys=Filt('MN_PSDAMP_P')  IC=[]
  Out : Outport
  wires:
  In/1 -> MN_PSDAMP_P/1
  MN_PSDAMP_P/1 -> Out/1

== system controlmodel/TypeA/Controller/MNservo/Damp_RMN ==
  In : Inport
  K1:VIS-OPTIC_MN_PSDAMP_R : LiveParts/LiveFilter  Tag=LiveFilter  par=Filt_MN_PSDAMP_R  prefix=['K1:VIS-',optic,'_MN_PSDAMP_R']  site='kamioka'  feModel=['K1VIS',optic,'P']  fmName=[optic,'_MN_PSDAMP_R']  flexTf=on  viewGui=off
      settings: AttributesFormatString=%<Tag>
  MN_PSDAMP_R : cstblocks/LTI System  sys=Filt('MN_PSDAMP_R')  IC=[]
  Out : Outport
  wires:
  In/1 -> MN_PSDAMP_R/1
  MN_PSDAMP_R/1 -> Out/1

== system controlmodel/TypeA/Controller/MNservo/Damp_TMN ==
  In : Inport
  K1:VIS-OPTIC_MN_PSDAMP_T : LiveParts/LiveFilter  Tag=LiveFilter  par=Filt_MN_PSDAMP_T  prefix=['K1:VIS-',optic,'_MN_PSDAMP_T']  site='kamioka'  feModel=['K1VIS',optic,'P']  fmName=[optic,'_MN_PSDAMP_T']  flexTf=on  viewGui=off
      settings: AttributesFormatString=%<Tag>
  MN_PSDAMP_T : cstblocks/LTI System  sys=Filt('MN_PSDAMP_T')  IC=[]
  Out : Outport
  wires:
  In/1 -> MN_PSDAMP_T/1
  MN_PSDAMP_T/1 -> Out/1

== system controlmodel/TypeA/Controller/MNservo/Damp_VMN ==
  In : Inport
  K1:VIS-OPTIC_MN_PSDAMP_V : LiveParts/LiveFilter  Tag=LiveFilter  par=Filt_MN_PSDAMP_V  prefix=['K1:VIS-',optic,'_MN_PSDAMP_V']  site='kamioka'  feModel=['K1VIS',optic,'P']  fmName=[optic,'_MN_PSDAMP_V']  flexTf=on  viewGui=off
      settings: AttributesFormatString=%<Tag>
  MN_PSDAMP_V : cstblocks/LTI System  sys=Filt('MN_PSDAMP_V')  IC=[]
  Out : Outport
  wires:
  In/1 -> MN_PSDAMP_V/1
  MN_PSDAMP_V/1 -> Out/1

== system controlmodel/TypeA/Controller/MNservo/Damp_YMN ==
  In : Inport
  K1:VIS-OPTIC_MN_PSDAMP_Y : LiveParts/LiveFilter  Tag=LiveFilter  par=Filt_MN_PSDAMP_Y  prefix=['K1:VIS-',optic,'_MN_PSDAMP_Y']  site='kamioka'  feModel=['K1VIS',optic,'P']  fmName=[optic,'_MN_PSDAMP_Y']  flexTf=on  viewGui=off
      settings: AttributesFormatString=%<Tag>
  MN_PSDAMP_Y : cstblocks/LTI System  sys=Filt('MN_PSDAMP_Y')  IC=[]
  Out : Outport
  wires:
  In/1 -> MN_PSDAMP_Y/1
  MN_PSDAMP_Y/1 -> Out/1

== system controlmodel/TypeA/Controller/MNservo/MNLOCK_L ==
  In : Inport
  K1:VIS-OPTIC_MN_LOCK_L : LiveParts/LiveFilter  Tag=LiveFilter  par=Filt_MN_LOCK_L  prefix=['K1:VIS-',optic,'_MN_LOCK_L']  site='kamioka'  feModel=['K1VIS',optic,'P']  fmName=[optic,'_MN_LOCK_L']  flexTf=on  viewGui=off
      settings: AttributesFormatString=%<Tag>
  MN_LOCK_L : cstblocks/LTI System  sys=Filt('MN_LOCK_L')  IC=[]
  Out : Outport
  wires:
  In/1 -> MN_LOCK_L/1
  MN_LOCK_L/1 -> Out/1

== system controlmodel/TypeA/Controller/MNservo/MNLOCK_P ==
  In : Inport
  K1:VIS-OPTIC_MN_LOCK_P : LiveParts/LiveFilter  Tag=LiveFilter  par=Filt_MN_LOCK_P  prefix=['K1:VIS-',optic,'_MN_LOCK_P']  site='kamioka'  feModel=['K1VIS',optic,'P']  fmName=[optic,'_MN_LOCK_P']  flexTf=on  viewGui=off
      settings: AttributesFormatString=%<Tag>
  MN_LOCK_P : cstblocks/LTI System  sys=Filt('MN_LOCK_P')  IC=[]
  Out : Outport
  wires:
  In/1 -> MN_LOCK_P/1
  MN_LOCK_P/1 -> Out/1

== system controlmodel/TypeA/Controller/MNservo/MNLOCK_Y ==
  In : Inport
  K1:VIS-OPTIC_MN_LOCK_Y : LiveParts/LiveFilter  Tag=LiveFilter  par=Filt_MN_LOCK_Y  prefix=['K1:VIS-',optic,'_MN_LOCK_Y']  site='kamioka'  feModel=['K1VIS',optic,'P']  fmName=[optic,'_MN_LOCK_Y']  flexTf=on  viewGui=off
      settings: AttributesFormatString=%<Tag>
  MN_LOCK_Y : cstblocks/LTI System  sys=Filt('MN_LOCK_Y')  IC=[]
  Out : Outport
  wires:
  In/1 -> MN_LOCK_Y/1
  MN_LOCK_Y/1 -> Out/1

== system controlmodel/TypeA/Controller/MNservo/OLDamp_PMN ==
  In : Inport
  K1:VIS-OPTIC_MN_MNOLDAMP_P : LiveParts/LiveFilter  Tag=LiveFilter  par=Filt_MN_MNOLDAMP_P  prefix=['K1:VIS-',optic,'_MN_MNOLDAMP_P']  site='kamioka'  feModel=['K1VIS',optic,'P']  fmName=[optic,'_MN_MNOLDAMP_P']  flexTf=on  viewGui=off
      settings: AttributesFormatString=%<Tag>
  MN_MNOLDAMP_P : cstblocks/LTI System  sys=Filt('MN_MNOLDAMP_P')  IC=[]
  Out : Outport
  wires:
  In/1 -> MN_MNOLDAMP_P/1
  MN_MNOLDAMP_P/1 -> Out/1

== system controlmodel/TypeA/Controller/MNservo/OLDamp_YMN ==
  In : Inport
  K1:VIS-OPTIC_MN_MNOLDAMP_Y : LiveParts/LiveFilter  Tag=LiveFilter  par=Filt_MN_MNOLDAMP_Y  prefix=['K1:VIS-',optic,'_MN_MNOLDAMP_Y']  site='kamioka'  feModel=['K1VIS',optic,'P']  fmName=[optic,'_MN_MNOLDAMP_Y']  flexTf=on  viewGui=off
      settings: AttributesFormatString=%<Tag>
  MN_MNOLDAMP_Y : cstblocks/LTI System  sys=Filt('MN_MNOLDAMP_Y')  IC=[]
  Out : Outport
  wires:
  In/1 -> MN_MNOLDAMP_Y/1
  MN_MNOLDAMP_Y/1 -> Out/1

== system controlmodel/TypeA/Controller/MNservo/TMOLDAMP_LMN ==
  In : Inport
  K1:VIS-OPTIC_MN_TMOLDAMP_L : LiveParts/LiveFilter  Tag=LiveFilter  par=Filt_MN_TMOLDAMP_L  prefix=['K1:VIS-',optic,'_MN_TMOLDAMP_L']  site='kamioka'  feModel=['K1VIS',optic,'P']  fmName=[optic,'_MN_TMOLDAMP_L']  flexTf=on  viewGui=off
      settings: AttributesFormatString=%<Tag>
  MN_TMOLDAMP_L : cstblocks/LTI System  sys=Filt('MN_TMOLDAMP_L')  IC=[]
  Out : Outport
  wires:
  In/1 -> MN_TMOLDAMP_L/1
  MN_TMOLDAMP_L/1 -> Out/1

== system controlmodel/TypeA/Controller/MNservo/TMOLDAMP_PMN ==
  In : Inport
  K1:VIS-OPTIC_MN_TMOLDAMP_P : LiveParts/LiveFilter  Tag=LiveFilter  par=Filt_MN_TMOLDAMP_P  prefix=['K1:VIS-',optic,'_MN_TMOLDAMP_P']  site='kamioka'  feModel=['K1VIS',optic,'P']  fmName=[optic,'_MN_TMOLDAMP_P']  flexTf=on  viewGui=off
      settings: AttributesFormatString=%<Tag>
  MN_TMOLDAMP_P : cstblocks/LTI System  sys=Filt('MN_TMOLDAMP_P')  IC=[]
  Out : Outport
  wires:
  In/1 -> MN_TMOLDAMP_P/1
  MN_TMOLDAMP_P/1 -> Out/1

== system controlmodel/TypeA/Controller/MNservo/TMOLDAMP_YMN ==
  In : Inport
  K1:VIS-OPTIC_MN_OLDAMP1_Y : LiveParts/LiveFilter  Tag=LiveFilter  par=Filt_MN_TMOLDAMP_Y  prefix=['K1:VIS-',optic,'_MN_TMOLDAMP_Y']  site='kamioka'  feModel=['K1VIS',optic,'P']  fmName=[optic,'_MN_TMOLDAMP_Y']  flexTf=on  viewGui=off
      settings: AttributesFormatString=%<Tag>
  MN_TMOLDAMP_Y : cstblocks/LTI System  sys=Filt('MN_TMOLDAMP_Y')  IC=[]
  Out : Outport
  wires:
  In/1 -> MN_TMOLDAMP_Y/1
  MN_TMOLDAMP_Y/1 -> Out/1

== system controlmodel/TypeA/Controller/TMservo/Damp_LTM ==
  In : Inport
  K1:VIS-OPTIC_TM_DAMP_L : LiveParts/LiveFilter  Tag=LiveFilter  par=Filt_TM_DAMP_L  prefix=['K1:VIS-',optic,'_TM_DAMP_L']  site='kamioka'  feModel=['K1VIS',optic,'P']  fmName=[optic,'_TM_DAMP_L']  flexTf=on  viewGui=off
      settings: AttributesFormatString=%<Tag>
  TM_DAMP_L : cstblocks/LTI System  sys=Filt('TM_DAMP_L')  IC=[]
  Out : Outport
  wires:
  In/1 -> TM_DAMP_L/1
  TM_DAMP_L/1 -> Out/1

== system controlmodel/TypeA/Controller/TMservo/Damp_PTM ==
  In : Inport
  K1:VIS-OPTIC_TM_DAMP_P : LiveParts/LiveFilter  Tag=LiveFilter  par=Filt_TM_DAMP_P  prefix=['K1:VIS-',optic,'_TM_DAMP_P']  site='kamioka'  feModel=['K1VIS',optic,'P']  fmName=[optic,'_TM_DAMP_P']  flexTf=on  viewGui=off
      settings: AttributesFormatString=%<Tag>
  TM_DAMP_P : cstblocks/LTI System  sys=Filt('TM_DAMP_P')  IC=[]
  Out : Outport
  wires:
  In/1 -> TM_DAMP_P/1
  TM_DAMP_P/1 -> Out/1

== system controlmodel/TypeA/Controller/TMservo/Damp_YTM ==
  In : Inport
  K1:VIS-OPTIC_TM_DAMP_Y : LiveParts/LiveFilter  Tag=LiveFilter  par=Filt_TM_DAMP_Y  prefix=['K1:VIS-',optic,'_TM_DAMP_Y']  site='kamioka'  feModel=['K1VIS',optic,'P']  fmName=[optic,'_TM_DAMP_Y']  flexTf=on  viewGui=off
      settings: AttributesFormatString=%<Tag>
  TM_DAMP_Y : cstblocks/LTI System  sys=Filt('TM_DAMP_Y')  IC=[]
  Out : Outport
  wires:
  In/1 -> TM_DAMP_Y/1
  TM_DAMP_Y/1 -> Out/1

== system controlmodel/TypeA/Controller/TMservo/LOCK_LTM ==
  In : Inport
  K1:VIS-OPTIC_TM_LOCK_L : LiveParts/LiveFilter  Tag=LiveFilter  par=Filt_TM_LOCK_L  prefix=['K1:VIS-',optic,'_TM_LOCK_L']  site='kamioka'  feModel=['K1VIS',optic,'P']  fmName=[optic,'_TM_LOCK_L']  flexTf=on  viewGui=off
      settings: AttributesFormatString=%<Tag>
  TM_LOCK_L : cstblocks/LTI System  sys=Filt('TM_LOCK_L')  IC=[]
  Out : Outport
  wires:
  In/1 -> TM_LOCK_L/1
  TM_LOCK_L/1 -> Out/1

== system controlmodel/TypeA/Controller/TMservo/LOCK_PTM ==
  In : Inport
  K1:VIS-OPTIC_TM_LOCK_P : LiveParts/LiveFilter  Tag=LiveFilter  par=Filt_TM_LOCK_P  prefix=['K1:VIS-',optic,'_TM_LOCK_P']  site='kamioka'  feModel=['K1VIS',optic,'P']  fmName=[optic,'_TM_LOCK_P']  flexTf=on  viewGui=off
      settings: AttributesFormatString=%<Tag>
  TM_LOCK_P : cstblocks/LTI System  sys=Filt('TM_LOCK_P')  IC=[]
  Out : Outport
  wires:
  In/1 -> TM_LOCK_P/1
  TM_LOCK_P/1 -> Out/1

== system controlmodel/TypeA/Controller/TMservo/LOCK_YTM ==
  In : Inport
  K1:VIS-OPTIC_TM_LOCK_Y : LiveParts/LiveFilter  Tag=LiveFilter  par=Filt_TM_LOCK_Y  prefix=['K1:VIS-',optic,'_TM_LOCK_Y']  site='kamioka'  feModel=['K1VIS',optic,'P']  fmName=[optic,'_TM_LOCK_Y']  flexTf=on  viewGui=off
      settings: AttributesFormatString=%<Tag>
  TM_LOCK_Y : cstblocks/LTI System  sys=Filt('TM_LOCK_Y')  IC=[]
  Out : Outport
  wires:
  In/1 -> TM_LOCK_Y/1
  TM_LOCK_Y/1 -> Out/1

== system controlmodel/TypeA/Controller/TMservo/SERVO_LTM ==
  In : Inport
  K1:VIS-OPTIC_TM_SERVO_L : LiveParts/LiveFilter  Tag=LiveFilter  par=Filt_TM_SERVO_L  prefix=['K1:VIS-',optic,'_TM_SERVO_L']  site='kamioka'  feModel=['K1VIS',optic,'P']  fmName=[optic,'_TM_SERVO_L']  flexTf=on  viewGui=off
      settings: AttributesFormatString=%<Tag>
  TM_SERVO_L : cstblocks/LTI System  sys=Filt('TM_SERVO_L')  IC=[]
  Out : Outport
  wires:
  In/1 -> TM_SERVO_L/1
  TM_SERVO_L/1 -> Out/1

== system controlmodel/TypeA/Controller/TMservo/SERVO_PTM ==
  In : Inport
  K1:VIS-OPTIC_TM_SERVO_P : LiveParts/LiveFilter  Tag=LiveFilter  par=Filt_TM_SERVO_P  prefix=['K1:VIS-',optic,'_TM_SERVO_P']  site='kamioka'  feModel=['K1VIS',optic,'P']  fmName=[optic,'_TM_SERVO_P']  flexTf=on  viewGui=off
      settings: AttributesFormatString=%<Tag>
  TM_SERVO_P : cstblocks/LTI System  sys=Filt('TM_SERVO_P')  IC=[]
  Out : Outport
  wires:
  In/1 -> TM_SERVO_P/1
  TM_SERVO_P/1 -> Out/1

== system controlmodel/TypeA/Controller/TMservo/SERVO_YTM ==
  In : Inport
  K1:VIS-OPTIC_TM_SERVO_Y : LiveParts/LiveFilter  Tag=LiveFilter  par=Filt_TM_SERVO_Y  prefix=['K1:VIS-',optic,'_TM_SERVO_Y']  site='kamioka'  feModel=['K1VIS',optic,'P']  fmName=[optic,'_TM_SERVO_Y']  flexTf=on  viewGui=off
      settings: AttributesFormatString=%<Tag>
  TM_SERVO_Y : cstblocks/LTI System  sys=Filt('TM_SERVO_Y')  IC=[]
  Out : Outport
  wires:
  In/1 -> TM_SERVO_Y/1
  TM_SERVO_Y/1 -> Out/1
